simulink model "task_G_mod"  (R2018a)
settings: Solver=ode4  StartTime=0.0  StopTime=10.0  FixedStep=0.01  RelTol=1e-3  EnableMultiTasking=on
values from neighbouring files (symbols this model uses):
  A = [0,1;-c/m,-beta/m]    [task_A_scr.m]    (also in task_B_scr.m = A*(16*lamda/(c*ro*h^2)); task_C1_scr.m = A*(16*lamda/(c*ro*h^2)); task_C_scr.m = A*(16*lamda/(c*ro*h^2)); task_D1_scr.m = A*(16*lamda/(c*ro*h^2)))
  B = [0;1]    [task_A_scr.m]    (also in task_B_scr.m = B*(4/(c*ro*h)); task_C1_scr.m = B*(4/(c*ro*h)); task_C_scr.m = B*(4/(c*ro*h)); task_D1_scr.m = B*(4/(c*ro*h)))
  C = [4/3,-1/3,0]    [task_C1_scr.m]    (also in task_C_scr.m; task_F1_scr.m; task_F_scr.m; task_G_scr.m)
  D = [h/(6*lamda),0]    [task_C1_scr.m]    (also in task_C_scr.m; task_F1_scr.m; task_F_scr.m; task_G_scr.m)
  nmax = 1.1    [task_E1_scr.m]    (also in task_E_scr.m; task_F1_scr.m; task_F_scr.m; task_G_scr.m)
  nmin = 0.9    [task_E1_scr.m]    (also in task_E_scr.m; task_F1_scr.m; task_F_scr.m; task_G_scr.m)
  nois = 1; sim('task_E1_mod',10)    [task_E1_scr.m]    (also in task_E_scr.m; task_F1_scr.m = 1; task_F_scr.m = 1; sim('task_F_mod',8); task_G_scr.m = 1; sim('task_G_mod',15))
  qa = 500000    [task_B_scr.m]    (also in task_C1_scr.m = 650000; task_C_scr.m; task_D1_scr.m = 550000; task_D2_scr.m)
  T_0 = 300    [task_B_scr.m]    (also in task_C1_scr.m; task_C_scr.m; task_D1_scr.m; task_D2_scr.m)
  Tb = 350    [task_B_scr.m]    (also in task_C1_scr.m = 403; sim('task_C1_mod',15); task_C_scr.m; task_D1_scr.m; task_D2_scr.m = 350; sim('task_D1_mod',10))
settings Model: Creator=Yurii  LastModifiedBy=Master
settings DataIOCC: LimitDataPoints=on  SaveFormat=Array
settings OptimizationCC: LifeSpan=inf
settings DebuggingCC: UnderspecifiedInitializationDetection=Classic  MergeDetectMultiDrivingBlocksExec=none  SolverPrmCheckMsg=warning  SFUnexpectedBacktrackingDiag=warning  SFNoUnconditionalDefaultTransitionDiag=warning  SFExecutionAtInitializationDiag=none
settings HardwareCC: ProdBitPerPointer=32  ProdBitPerSizeT=32  ProdBitPerPtrDiffT=32  ProdLargestAtomicFloat=None  ProdIntDivRoundTo=Undefined  ProdEndianess=Unspecified  ProdWordSize=32  ProdHWDeviceType=32-bit Generic
settings ModelReferenceCC: PropagateSignalLabelsOutOfModel=off
settings CodeAppCC: StateflowObjectComments=on
settings GRTTargetCC: TargetLangStandard=C89/C90 (ANSI)  GeneratePreprocessorConditionals=Disable all
settings ConfigComp: CovMetricSettings=dw  CovHtmlReporting=on  CovSaveCumulativeToWorkspaceVar=on  CovSaveSingleToWorkspaceVar=on  CovExternalEMLEnable=off

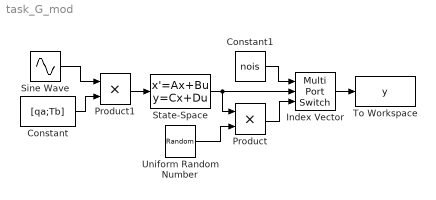
== system task_G_mod ==
  Constant : Constant  Value=[qa;Tb]
  Constant1 : Constant  Value=nois
  Index Vector : MultiPortSwitch  DataPortOrder=Zero-based contiguous  Inputs=2  zeroidx=on
  Product : Product
  Product1 : Product
  Sine Wave : Sin  Amplitude=0.01  Bias=1  SampleTime=0
  State-Space : StateSpace  A=A  B=B  C=C  D=D  InitialCondition=[T_0;T_0;T_0]
  To Workspace : ToWorkspace  VariableName=y  SaveFormat=Timeseries  SampleTime=-1
  Uniform Random Number : UniformRandomNumber  Minimum=nmin  Maximum=nmax  SampleTime=0
  wires:
  Uniform Random Number/1 -> Product/2
  State-Space/1 -> Product/1, Index Vector/2
  Product/1 -> Index Vector/3
  Index Vector/1 -> To Workspace/1
  Constant1/1 -> Index Vector/1
  Product1/1 -> State-Space/1
  Constant/1 -> Product1/2
  Sine Wave/1 -> Product1/1
